simulink model "string_dynamics"  (R2023b)
settings: Solver=ode8  StartTime=0.0  StopTime=2000  FixedStep=.1  RelTol=1e-3
undefined symbols (not defined in the file): ic, p
settings Model: Creator=cyrus  LastModifiedBy=cyrus

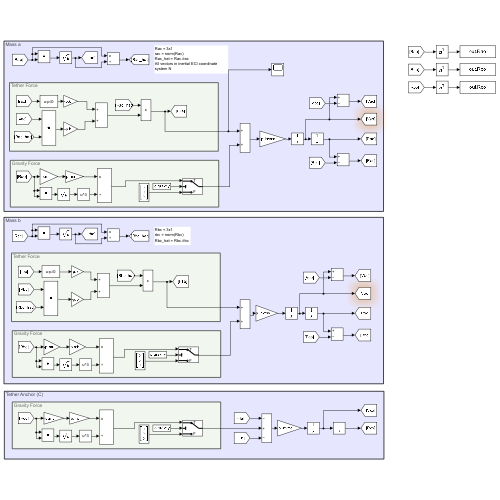
[thumbnail: Simulink's stored preview of the top-level diagram]
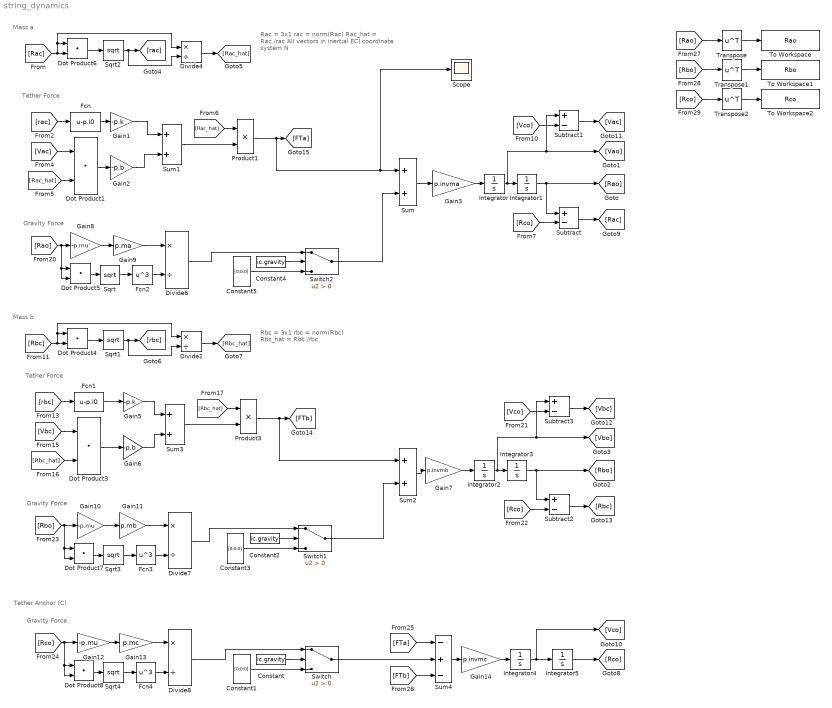
== system string_dynamics ==
  note: Gravity Force
  note: Tether Anchor (C)
  note: Tether Force
  note: Rac = 3x1
      | rac = norm(Rac)
      | Rac_hat = Rac./rac
      | All vectors in inertial ECI coordinate system N
  note: Mass a
  note: Rbc = 3x1
      | rbc = norm(Rbc)
      | Rbc_hat = Rbc./rbc
  note: Tether Force
  note: Mass b
  note: Gravity Force
  note: Gravity Force
  Constant : Constant  Value=ic.gravity
  Constant1 : Constant  Value=[0;0;0]  VectorParams1D=off
  Constant2 : Constant  Value=ic.gravity
  Constant3 : Constant  Value=[0;0;0]  VectorParams1D=off
  Constant4 : Constant  Value=ic.gravity
  Constant5 : Constant  Value=[0;0;0]  VectorParams1D=off
  Divide{2,4,6..8} (5 alike) : Product  Inputs=*/
  Dot Product{1,3..8} (7 alike) : DotProduct  OutDataTypeStr=Inherit: Inherit via internal rule
  Fcn : Fcn  Expr=u-p.l0
  Fcn1 : Fcn  Expr=u-p.l0
  Fcn2 : Fcn  Expr=u^3
  Fcn3 : Fcn  Expr=u^3
  Fcn4 : Fcn  Expr=u^3
  Gain1 : Gain  Gain=-p.k
  Gain10 : Gain  Gain=-p.mu
  Gain11 : Gain  Gain=p.mb
  Gain12 : Gain  Gain=-p.mu
  Gain13 : Gain  Gain=p.mc
  Gain14 : Gain  Gain=p.invmc
  Gain2 : Gain  Gain=-p.b
  Gain3 : Gain  Gain=p.invma
  Gain5 : Gain  Gain=-p.k
  Gain6 : Gain  Gain=-p.b
  Gain7 : Gain  Gain=p.invmb
  Gain8 : Gain  Gain=-p.mu'
  Gain9 : Gain  Gain=p.ma
  Integrator : Integrator  InitialCondition=ic.NVao0
  Integrator1 : Integrator  InitialCondition=ic.NRao0
  Integrator2 : Integrator  InitialCondition=ic.NVbo0
  Integrator3 : Integrator  InitialCondition=ic.NRbo0
  Integrator4 : Integrator  InitialCondition=ic.NVco0
  Integrator5 : Integrator  InitialCondition=ic.NRco0
  Product1 : Product
  Product3 : Product
  Scope : Scope
  Sqrt{,1..4} (5 alike) : Sqrt
  Subtract{,1..3} (4 alike) : Sum  Inputs=+-
  Sum{,1..3} (4 alike) : Sum
  Sum4 : Sum  Inputs=-+-
  Switch : Switch  Criteria=u2 > Threshold  SaturateOnIntegerOverflow=off  InputSameDT=off
  Switch1 : Switch  Criteria=u2 > Threshold  SaturateOnIntegerOverflow=off  InputSameDT=off
  Switch2 : Switch  Criteria=u2 > Threshold  SaturateOnIntegerOverflow=off  InputSameDT=off
  To Workspace : ToWorkspace  VariableName=Rao  SampleTime=-1
      settings: Save2DSignal=2-D array (concatenate along first dimension)
  To Workspace1 : ToWorkspace  VariableName=Rbo  SampleTime=-1
      settings: Save2DSignal=2-D array (concatenate along first dimension)
  To Workspace2 : ToWorkspace  VariableName=Rco  SampleTime=-1
      settings: Save2DSignal=2-D array (concatenate along first dimension)
  Transpose : Math  Operator=transpose
  Transpose1 : Math  Operator=transpose
  Transpose2 : Math  Operator=transpose
  wires:
  [Rac] -> Divide4/1, Dot Product6/1, Dot Product6/2
  Dot Product6/1 -> Sqrt2/1
  Sqrt2/1 -> Divide4/2, [rac]
  Divide4/1 -> [Rac_hat]
  [rac] -> Fcn/1
  Fcn/1 -> Gain1/1
  Gain1/1 -> Sum1/1
  [Vac] -> Dot Product1/1
  [Rac_hat] -> Dot Product1/2
  Dot Product1/1 -> Gain2/1
  Gain2/1 -> Sum1/2
  [Rac_hat] -> Product1/1
  Sum1/1 -> Product1/2
  Sum/1 -> Gain3/1
  Gain3/1 -> Integrator/1
  Integrator/1 -> Integrator1/1, Subtract1/1, [Vao]
  Integrator1/1 -> Subtract/1, [Rao]
  [Rbc_hat] -> Dot Product3/2
  Sum3/1 -> Product3/2
  [rbc] -> Fcn1/1
  Divide2/1 -> [Rbc_hat]
  Sqrt1/1 -> Divide2/2, [rbc]
  Gain5/1 -> Sum3/1
  Fcn1/1 -> Gain5/1
  [Vbc] -> Dot Product3/1
  Sum2/1 -> Gain7/1
  Gain6/1 -> Sum3/2
  Dot Product4/1 -> Sqrt1/1
  [Rbc_hat] -> Product3/1
  Dot Product3/1 -> Gain6/1
  [Rbc] -> Divide2/1, Dot Product4/1, Dot Product4/2
  [Rco] -> Subtract/2
  Subtract/1 -> [Rac]
  [Vco] -> Subtract1/2
  Subtract1/1 -> [Vac]
  [Rao] -> Dot Product5/2, Dot Product5/1, Gain8/1
  Gain8/1 -> Gain9/1
  Gain9/1 -> Divide6/1
  Fcn2/1 -> Divide6/2
  Sqrt/1 -> Fcn2/1
  Dot Product5/1 -> Sqrt/1
  Integrator2/1 -> Integrator3/1, Subtract3/1, [Vbo]
  [Vco] -> Subtract3/2
  Subtract3/1 -> [Vbc]
  Gain7/1 -> Integrator2/1
  [Rco] -> Subtract2/2
  Integrator3/1 -> Subtract2/1, [Rbo]
  Subtract2/1 -> [Rbc]
  Gain10/1 -> Gain11/1
  Fcn3/1 -> Divide7/2
  Sqrt3/1 -> Fcn3/1
  Dot Product7/1 -> Sqrt3/1
  [Rbo] -> Dot Product7/2, Dot Product7/1, Gain10/1
  Gain11/1 -> Divide7/1
  Gain13/1 -> Divide8/1
  [Rco] -> Dot Product8/2, Dot Product8/1, Gain12/1
  Sqrt4/1 -> Fcn4/1
  Fcn4/1 -> Divide8/2
  Dot Product8/1 -> Sqrt4/1
  Gain12/1 -> Gain13/1
  Gain14/1 -> Integrator4/1
  Integrator4/1 -> [Vco], Integrator5/1
  Sum4/1 -> Gain14/1
  Integrator5/1 -> [Rco]
  [FTa] -> Sum4/1
  [FTb] -> Sum4/3
  Product3/1 -> Sum2/1, [FTb]
  Product1/1 -> Scope/1, Sum/1, [FTa]
  Switch/1 -> Sum4/2
  [Rao] -> Transpose/1
  Transpose/1 -> To Workspace/1
  [Rbo] -> Transpose1/1
  Transpose1/1 -> To Workspace1/1
  [Rco] -> Transpose2/1
  Transpose2/1 -> To Workspace2/1
  Constant/1 -> Switch/2
  Divide8/1 -> Switch/1
  Constant1/1 -> Switch/3
  Constant2/1 -> Switch1/2
  Constant3/1 -> Switch1/3
  Divide7/1 -> Switch1/1
  Constant4/1 -> Switch2/2
  Constant5/1 -> Switch2/3
  Divide6/1 -> Switch2/1
  Switch1/1 -> Sum2/2
  Switch2/1 -> Sum/2
